simulink model "Phase_Shift_Control_Model_No_DeadTime_V1_0"  (R2016b)
settings: Solver=VariableStepAuto  StartTime=0.0  StopTime=5/100000  RelTol=1e-3
libraries: simulink_extras x2
settings Model: Creator=whl14  LastModifiedBy=whl14

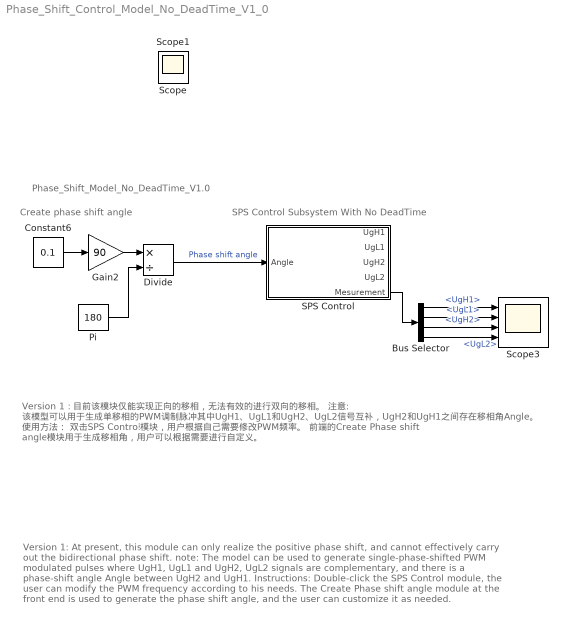
== system Phase_Shift_Control_Model_No_DeadTime_V1_0 ==
  note: Phase_Shift_Model_No_DeadTime_V1.0
  note: Version 1:
      | At present, this module can only realize the positive phase shift, and cannot effectively carry out the bidirectional phase shift.
      | note:
      | The model can be used to generate single-phase-shifted PWM modulated pulses where UgH1, UgL1 and UgH2, UgL2 signals are complementary, and there is a phase-shift angle Angle between UgH2 and UgH1.
      | Instructions:
      | Double-click the SPS Control module, the user can modify the PWM frequency according to his needs.
      | The Create Phase shift angle module at the front end is used to generate the phase shift angle, and the user can customize it as needed.
  note: Version 1 :
      | 目前该模块仅能实现正向的移相，无法有效的进行双向的移相。
      | 注意:
      | 该模型可以用于生成单移相的PWM调制脉冲其中UgH1、UgL1和UgH2、UgL2信号互补，UgH2和UgH1之间存在移相角Angle。
      | 使用方法：
      | 双击SPS Control模块，用户根据自己需要修改PWM频率。
      | 前端的Create Phase shift angle模块用于生成移相角，用户可以根据需要进行自定义。
  note: Create phase shift angle
  note: SPS Control Subsystem With No DeadTime
  Bus Selector : BusSelector  OutputSignals=UgH1,UgL1,UgH2,UgL2
  Constant6 : Constant  Value=0.1
  Divide : Product  Inputs=*/
  Gain2 : Gain  Gain=90
  Pi : Constant  Value=180
  SPS Control : Subsystem  mask(SPS Control SubModel description){fs=100000}
      mask help:
      | Define the frequency about the PWM, double clik the subsystem 'SPS Control' and change the value about the fs
      |
      | The input signal is a phase shift angle, which can be defined by the user as required
      mask Display: disp('SPS control')
  Scope3 : Scope  NumInputPorts=4
  Scope : Scope
  Scope1 : Scope
  wires:
  SPS Control/5(Mesurement) -> Bus Selector/1
  Bus Selector/1 -> Scope3/1  "<UgH1>"
  Bus Selector/2 -> Scope3/2  "<UgL1>"
  Bus Selector/3 -> Scope3/3  "<UgH2>"
  Bus Selector/4 -> Scope3/4  "<UgL2>"
  Gain2/1 -> Divide/1
  Constant6/1 -> Gain2/1
  Pi/1 -> Divide/2
  Divide/1 -> SPS Control/1(Angle)  "Phase shift angle"

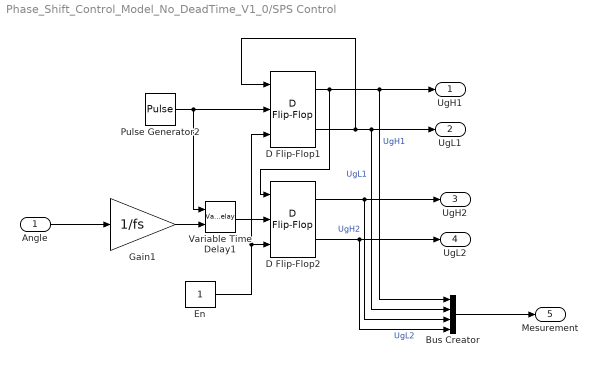
== system Phase_Shift_Control_Model_No_DeadTime_V1_0/SPS Control ==
  Angle : Inport
  Bus Creator : BusCreator  Inputs=4
  D Flip-Flop1 : simulink_extras/Flip Flops/D Flip-Flop
  D Flip-Flop2 : simulink_extras/Flip Flops/D Flip-Flop
  En : Constant
  Gain1 : Gain  Gain=1/fs
  Pulse Generator2 : DiscretePulseGenerator  PulseType=Time based  Period=1/(2*fs)  PulseWidth=50  VectorParams1D=off
  Variable Time Delay1 : VariableTransportDelay  MaximumDelay=10  ZeroDelay=on
  UgH1 : Outport
  UgL1 : Outport  Port=2
  UgH2 : Outport  Port=3
  UgL2 : Outport  Port=4
  Mesurement : Outport  Port=5
  wires:
  D Flip-Flop2/2 -> Bus Creator/4, UgL2/1  "UgL2"
  D Flip-Flop1/2 -> Bus Creator/2, UgL1/1, D Flip-Flop1/1  "UgL1"
  D Flip-Flop2/1 -> Bus Creator/3, UgH2/1  "UgH2"
  Gain1/1 -> Variable Time Delay1/2
  Variable Time Delay1/1 -> D Flip-Flop2/2
  En/1 -> D Flip-Flop1/3, D Flip-Flop2/3
  Pulse Generator2/1 -> D Flip-Flop1/2, Variable Time Delay1/1
  D Flip-Flop1/1 -> Bus Creator/1, UgH1/1, D Flip-Flop2/1  "UgH1"
  Angle/1 -> Gain1/1
  Bus Creator/1 -> Mesurement/1
